simulink model "mrac_2vars_linear_maglev"  (R2018a)
settings: Solver=VariableStepAuto  StartTime=0.0  StopTime=100  MaxStep=1e-2  RelTol=1e-3
InitFcn:
  | b0 = 12;
  | b1 = 6;
  | a0 = 20;
settings Model: Creator=saad  LastModifiedBy=saad

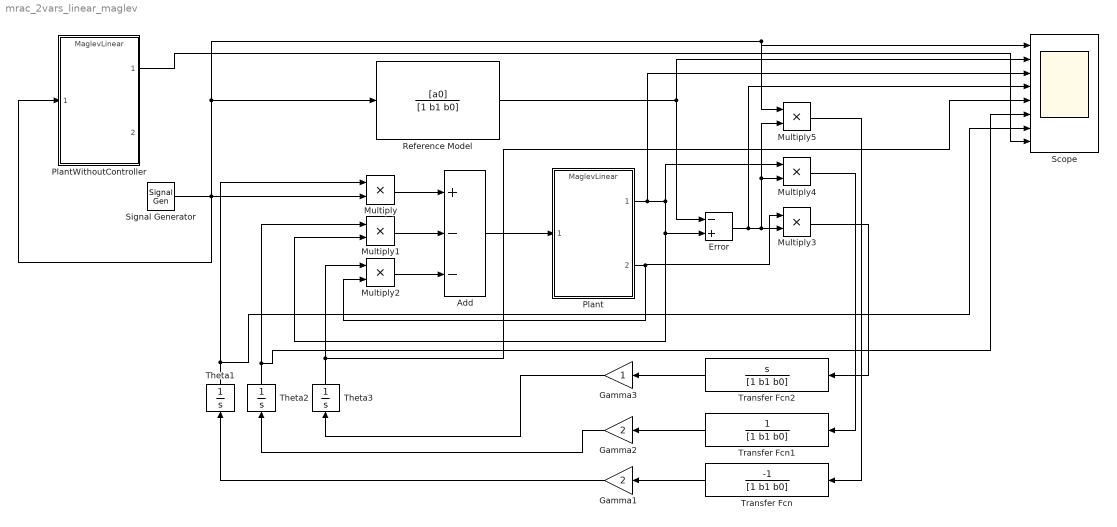
== system mrac_2vars_linear_maglev ==
  Add : Sum  Inputs=+--
  Error : Sum  Inputs=-+
  Gamma1 : Gain  Gain=2
  Gamma2 : Gain  Gain=2
  Gamma3 : Gain
  Multiply{,1..5} (6 alike) : Product
  Plant : ModelReference  ModelNameDialog=MaglevLinear  SimulationMode=Normal  ModelReferenceVersion=1.3
  PlantWithoutController : ModelReference  ModelNameDialog=MaglevLinear  SimulationMode=Normal  ModelReferenceVersion=1.3
  Reference Model : TransferFcn  Numerator=[a0]  Denominator=[1 b1 b0]
  Scope : Scope  NumInputPorts=8
  Signal Generator : SignalGenerator  WaveForm=square  Frequency=0.1
  Theta1 : Integrator
  Theta2 : Integrator
  Theta3 : Integrator
  Transfer Fcn : TransferFcn  Numerator=[-1]  Denominator=[1 b1 b0]
  Transfer Fcn1 : TransferFcn  Denominator=[1 b1 b0]
  Transfer Fcn2 : TransferFcn  Numerator=[1 0]  Denominator=[1 b1 b0]
  wires:
  Signal Generator/1 -> PlantWithoutController/1, Multiply5/1, Scope/1, Reference Model/1, Multiply/2
  Theta1/1 -> Scope/7, Multiply/1
  Theta2/1 -> Scope/6, Multiply1/1
  Theta3/1 -> Scope/5, Multiply2/1
  Multiply/1 -> Add/1
  Multiply1/1 -> Add/2
  Multiply2/1 -> Add/3
  Add/1 -> Plant/1
  Plant/1 -> Scope/3, Error/2, Multiply1/2, Multiply4/1
  Plant/2 -> Multiply3/1, Multiply2/2
  Reference Model/1 -> Scope/2, Error/1
  Error/1 -> Scope/4, Multiply5/2, Multiply4/2, Multiply3/2
  Multiply3/1 -> Transfer Fcn2/1
  Multiply4/1 -> Transfer Fcn1/1
  Multiply5/1 -> Transfer Fcn/1
  Transfer Fcn2/1 -> Gamma3/1
  Transfer Fcn1/1 -> Gamma2/1
  Transfer Fcn/1 -> Gamma1/1
  Gamma1/1 -> Theta1/1
  Gamma2/1 -> Theta2/1
  Gamma3/1 -> Theta3/1
  PlantWithoutController/1 -> Scope/8
